simulink model "VTLD_5"  (R2018a)
settings: Solver=VariableStepAuto  StartTime=0.0  StopTime=4  RelTol=1e-3
libraries: powerlib x12, powerlib_meascontrol x1
settings Model: Creator=Rafael Pavan  LastModifiedBy=Rafael Pavan

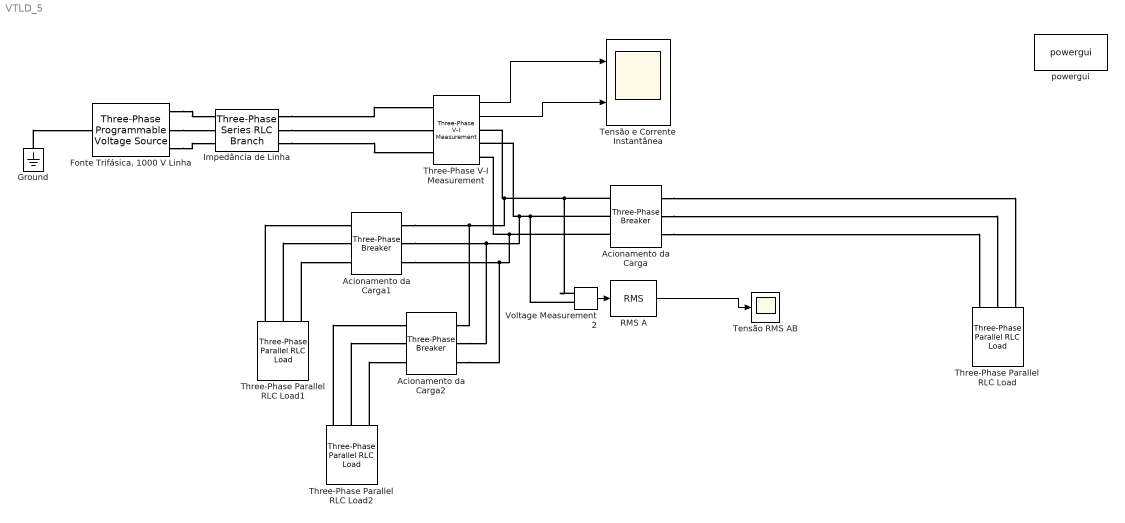
== system VTLD_5 ==
  Acionamento da Carga : powerlib/Elements/Three-Phase Breaker  InitialState=open  SwitchA=on  SwitchB=off  SwitchC=off  SwitchTimes=[0.4 300]  External=off  BreakerResistance=0.01  SnubberResistance=1e6  SnubberCapacitance=inf  Measurements=None
  Acionamento da Carga1 : powerlib/Elements/Three-Phase Breaker  InitialState=open  SwitchA=on  SwitchB=off  SwitchC=off  SwitchTimes=[0.7 300]  External=off  BreakerResistance=0.01  SnubberResistance=1e6  SnubberCapacitance=inf  Measurements=None
  Acionamento da Carga2 : powerlib/Elements/Three-Phase Breaker  InitialState=open  SwitchA=on  SwitchB=off  SwitchC=off  SwitchTimes=[0.9 300]  External=off  BreakerResistance=0.01  SnubberResistance=1e6  SnubberCapacitance=inf  Measurements=None
  "Fonte Trifásica, 1000 V Linha " : powerlib/Electrical Sources/Three-Phase Programmable Voltage Source  PositiveSequence=[1000 0 60]  VariationEntity=None  VariationType=Table of time-amplitude pairs  VariationTypeAlt=Step  VariationStep=0.5  VariationRate=10  VariationMagnitude=0.3  VariationFrequency=2  VariationTiming=[1 2]  VariationPhaseA=off  Amplitudes=[1 0.8 1.2 1.0]  TimeValues=[0 0.1 0.15 0.2]  HarmonicGeneration=off  HarmonicA=[3 0.2 -25 0]  HarmonicB=[2 0.15 35 2]  Timing="[0.05  3]"  BusType=PV  Pref=1000000000  Qref=0  Qmin=-inf  Qmax=inf
  Ground : powerlib/Elements/Ground  LConnTagsString=a
  "Impedância de Linha " : powerlib/Elements/Three-Phase Series RLC Branch  LConnTagsString=A|B|C  RConnTagsString=A|B|C  BranchType=RL  Resistance=0.01  Inductance=1e-3  Capacitance=1e-2  Measurements=None
  "RMS A " : powerlib_meascontrol/Measurements/RMS  TrueRMS=on  Freq=60  RMSInit=1000  Ts=0
  "Tensão RMS AB " : Scope
  Tensão e Corrente Instantânea : Scope  NumInputPorts=2
  Three-Phase Parallel RLC Load : powerlib/Elements/Three-Phase Parallel RLC Load  LConnTagsString=A|B|C  Configuration=Y (grounded)  NominalVoltage=1000  Vabc=[1e3 1e3 1e3]  Vabcp=[1e3 1e3 1e3]  NominalFrequency=60  UnbalancedPower=off  ActivePower=20000  InductivePower=0  CapacitivePower=0  Pabc=[10e3 9e3 11e3]  QLabc=[100 90 110]  QCabc=[100 90 110]  Pabcp=[10e3 9e3 11e3]  QLabcp=[100 90 110]  QCabcp=[100 90 110]  Measurements=None  LoadType=constant Z
  Three-Phase Parallel RLC Load1 : powerlib/Elements/Three-Phase Parallel RLC Load  LConnTagsString=A|B|C  Configuration=Y (grounded)  NominalVoltage=1000  Vabc=[1e3 1e3 1e3]  Vabcp=[1e3 1e3 1e3]  NominalFrequency=60  UnbalancedPower=off  ActivePower=1000  InductivePower=10000  CapacitivePower=12000  Pabc=[10e3 9e3 11e3]  QLabc=[100 90 110]  QCabc=[100 90 110]  Pabcp=[10e3 9e3 11e3]  QLabcp=[100 90 110]  QCabcp=[100 90 110]  Measurements=None  LoadType=constant Z
  Three-Phase Parallel RLC Load2 : powerlib/Elements/Three-Phase Parallel RLC Load  LConnTagsString=A|B|C  Configuration=Y (grounded)  NominalVoltage=1000  Vabc=[1e3 1e3 1e3]  Vabcp=[1e3 1e3 1e3]  NominalFrequency=60  UnbalancedPower=off  ActivePower=800000  InductivePower=10000  CapacitivePower=12000  Pabc=[10e3 9e3 11e3]  QLabc=[100 90 110]  QCabc=[100 90 110]  Pabcp=[10e3 9e3 11e3]  QLabcp=[100 90 110]  QCabcp=[100 90 110]  Measurements=None  LoadType=constant Z
  Three-Phase V-I Measurement : powerlib/Measurements/Three-Phase V-I Measurement  VoltageMeasurement=phase-to-phase  SetLabelV=off  LabelV=Vabc  Vpu=off  VpuLL=off  CurrentMeasurement=yes  SetLabelI=off  LabelI=Iabc  Ipu=off  Pbase=100e6  Vbase=220  OutputType=Complex  PhasorSimulation=off  PSBequivalent=0
  Voltage Measurement2 : powerlib/Measurements/Voltage Measurement  PhasorSimulation=off  OutputType=Complex  PSBequivalent=0
  powergui : powerlib/powergui  Priority=1  SimulationMode=Continuous  SampleTime=50e-6  frequency=60  Iterations=50  frequencyindice=60  Pbase=100e6  ErrMax=1e-4  UnitsV=kV  UnitsW=MW  buscounter=0  FunctionMessages=on  echomessages=off  EnableUseOfTLC=off  CurrentSourceSwitches=off  DisableSnubberDevices=off  DisableRonSwitches=off  DisableVfSwitches=off  DisplayEquations=off  SolverType=Tustin/Backward Euler (TBE)  Interpol=off  ExternalGateDelay=off  methode=off  Ts=100  x0status=blocks  SPID=on  SwTol=0  HookPort=off  RestoreLinks=warning  ResistiveCurrentMeasurement=off  Frange=[0:2:500]  Ylog=off  Xlog=on  ShowGrid=off  save=off  variable=ZData  structure=0  ZoomFFT=off  StartTime=0.0  cycles=1  DisplayStyle=1  fundamental=60  FreqAxis=off  MaxFrequency=1000  frequencyindicesteady=1  RmsSteady=1  display=off
  wires:
  Three-Phase V-I Measurement/2 -> Tensão e Corrente Instantânea/2
  Three-Phase V-I Measurement/1 -> Tensão e Corrente Instantânea/1
  "RMS A "/1 -> "Tensão RMS AB "/1
  Voltage Measurement2/1 -> "RMS A "/1
  connections:
  "Fonte Trifásica, 1000 V Linha "/RConn1 -- "Impedância de Linha "/LConn1
  "Fonte Trifásica, 1000 V Linha "/RConn2 -- "Impedância de Linha "/LConn2
  "Fonte Trifásica, 1000 V Linha "/RConn3 -- "Impedância de Linha "/LConn3
  "Impedância de Linha "/RConn2 -- Three-Phase V-I Measurement/LConn2
  "Impedância de Linha "/RConn1 -- Three-Phase V-I Measurement/LConn1
  "Impedância de Linha "/RConn3 -- Three-Phase V-I Measurement/LConn3
  Acionamento da Carga/LConn1 -- Voltage Measurement2/LConn1 -- Acionamento da Carga2/RConn1 -- Acionamento da Carga1/RConn1 -- Three-Phase V-I Measurement/RConn1
  Acionamento da Carga/LConn2 -- Voltage Measurement2/LConn2 -- Acionamento da Carga2/RConn2 -- Acionamento da Carga1/RConn2 -- Three-Phase V-I Measurement/RConn2
  Acionamento da Carga/LConn3 -- Acionamento da Carga2/RConn3 -- Acionamento da Carga1/RConn3 -- Three-Phase V-I Measurement/RConn3
  Ground/LConn1 -- "Fonte Trifásica, 1000 V Linha "/LConn1
  Acionamento da Carga/RConn3 -- Three-Phase Parallel RLC Load/LConn1
  Acionamento da Carga/RConn2 -- Three-Phase Parallel RLC Load/LConn2
  Acionamento da Carga/RConn1 -- Three-Phase Parallel RLC Load/LConn3
  Three-Phase Parallel RLC Load1/LConn3 -- Acionamento da Carga1/LConn3
  Three-Phase Parallel RLC Load1/LConn2 -- Acionamento da Carga1/LConn2
  Three-Phase Parallel RLC Load1/LConn1 -- Acionamento da Carga1/LConn1
  Three-Phase Parallel RLC Load2/LConn3 -- Acionamento da Carga2/LConn3
  Three-Phase Parallel RLC Load2/LConn2 -- Acionamento da Carga2/LConn2
  Three-Phase Parallel RLC Load2/LConn1 -- Acionamento da Carga2/LConn1
